simulink model "task_2"  (R2021b)
settings: Solver=VariableStepAuto  StartTime=0.0  StopTime=t  MaxStep=1e-2  RelTol=1e-3
values from neighbouring files (symbols this model uses):
  a1 = -4    [env_practice_2.m]
  a2 = -1.6    [env_practice_2.m]
  adapt_control = 1    [env_practice_2.m]
  am1 = -100/9    (= -11.1111111111)    [env_practice_2.m]
  am2 = -50/9    (= -5.55555555556)    [env_practice_2.m]
  b = 8    [env_practice_2.m]
  bm = 300/9    (= 33.3333333333)    [env_practice_2.m]
  ga = ga.*100    [env_practice_2.m]
  gb = gb*100    (= 100)    [env_practice_2.m]
  P = [1.34 0.045; 0.045 0.0981]    [env_practice_2.m]
  pulse = 1    [env_practice_2.m]
undefined symbols (not defined in the file or in its folder): au, bu, ga1, ga2
settings Model: Creator=79159  LastModifiedBy=79159

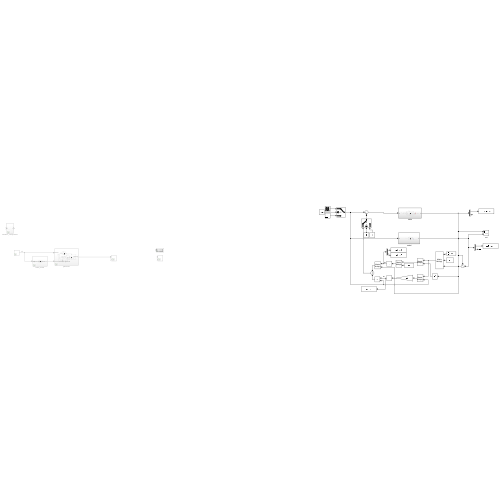
[thumbnail: Simulink's stored preview of the top-level diagram]
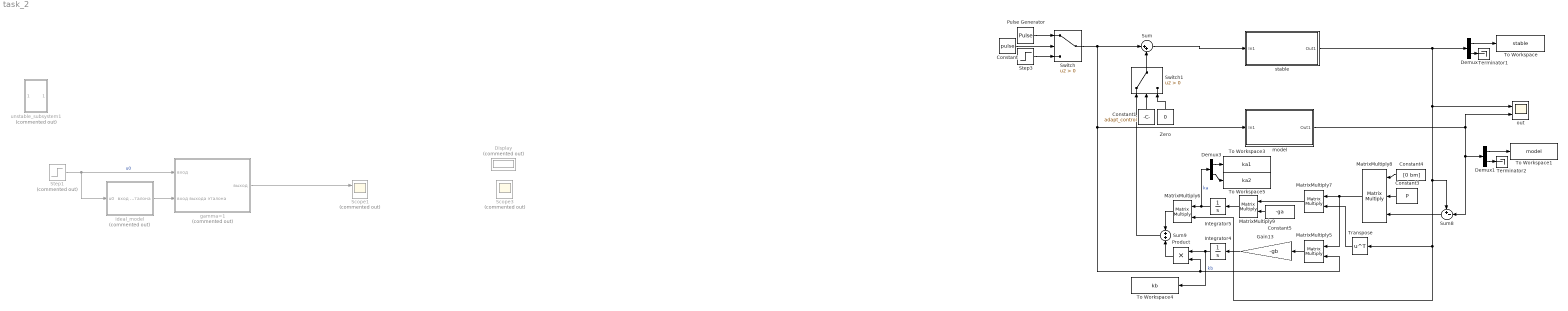
== system task_2 ==
  Constant : Constant  Value=pulse
  Constant1 : Constant  Value=adapt_control
  Constant3 : Constant  Value=P  VectorParams1D=off
  Constant4 : Constant  Value=[0 bm]  VectorParams1D=off
  Constant5 : Constant  Value=-ga  VectorParams1D=off
  Demux : Demux  Outputs=2
  Demux1 : Demux  Outputs=2
  Demux3 : Demux  Outputs=2
  Display : Display  Commented=on
      settings: Decimation=2
  Gain13 : Gain  Gain=-gb
  Integrator4 : Integrator
  Integrator5 : Integrator
  MatrixMultiply{5..7,9} (4 alike) : Product  Multiplication=Matrix(*)
  MatrixMultiply8 : Product  Inputs=3  Multiplication=Matrix(*)
  Product : Product
  Pulse Generator : DiscretePulseGenerator  PulseType=Time based  Period=20  PulseWidth=50
  Scope1 : Scope  Commented=on  NumInputPorts=2
  Scope3 : Scope  Commented=on  NumInputPorts=2
  Step1 : Step  Commented=on  Time=0  SampleTime=0
  Step3 : Step  Time=0  SampleTime=0
  Sum : Sum  Inputs=|++
  Sum8 : Sum  Inputs=+-|
  Sum9 : Sum  Inputs=+|+
  Switch : Switch  Criteria=u2 > Threshold
  Switch1 : Switch  Criteria=u2 > Threshold
  Terminator1 : Terminator
  Terminator2 : Terminator
  To Workspace : ToWorkspace  VariableName=stable  SaveFormat=Timeseries  SampleTime=-1
  To Workspace1 : ToWorkspace  VariableName=model  SaveFormat=Timeseries  SampleTime=-1
  To Workspace3 : ToWorkspace  VariableName=ka1  SaveFormat=Timeseries  SampleTime=-1
  To Workspace4 : ToWorkspace  VariableName=kb  SaveFormat=Timeseries  SampleTime=-1
  To Workspace5 : ToWorkspace  VariableName=ka2  SaveFormat=Timeseries  SampleTime=-1
  Transpose : Math  Operator=transpose  SaturateOnIntegerOverflow=on
  Zero : Constant  Value=0  OutDataTypeStr=Inherit: Inherit via back propagation
  gamma=1 : Subsystem  Commented=on
  ideal_model : Subsystem  Commented=on
  model : Subsystem
  out : Scope  NumInputPorts=2
  stable : Subsystem
  unstable_subsystem1 : Subsystem  Commented=on
  wires:
  Step1/1 -> ideal_model/1(u0), gamma=1/1(вход)  "u0"
  ideal_model/1(вход выхода эталона) -> gamma=1/2(вход выхода эталона)
  gamma=1/1(выход) -> Scope1/1
  Switch/1 -> model/1(In1), Product/2, MatrixMultiply5/2, Sum/1
  Product/1 -> Sum9/2
  stable/1(Out1) -> Demux/1, out/1, Sum8/1, Transpose/1, MatrixMultiply6/2
  MatrixMultiply7/1 -> MatrixMultiply9/1
  Sum8/1 -> MatrixMultiply8/3
  MatrixMultiply8/1 -> MatrixMultiply5/1, MatrixMultiply7/1
  Constant5/1 -> MatrixMultiply9/2
  Constant4/1 -> MatrixMultiply8/1
  Constant3/1 -> MatrixMultiply8/2
  Integrator5/1 -> Demux3/1, MatrixMultiply6/1  "ka"
  MatrixMultiply6/1 -> Sum9/1
  Gain13/1 -> Integrator4/1
  Transpose/1 -> MatrixMultiply7/2
  MatrixMultiply9/1 -> Integrator5/1
  MatrixMultiply5/1 -> Gain13/1
  Integrator4/1 -> To Workspace4/1, Product/1  "kb"
  Sum/1 -> stable/1(In1)
  model/1(Out1) -> Demux1/1, Sum8/2, out/2
  Demux/1 -> To Workspace/1
  Demux1/1 -> To Workspace1/1
  Demux3/1 -> To Workspace3/1
  Demux3/2 -> To Workspace5/1
  Demux/2 -> Terminator1/1
  Demux1/2 -> Terminator2/1
  Pulse Generator/1 -> Switch/1
  Step3/1 -> Switch/3
  Constant/1 -> Switch/2
  Sum9/1 -> Switch1/1
  Constant1/1 -> Switch1/2
  Switch1/1 -> Sum/2
  Zero/1 -> Switch1/3

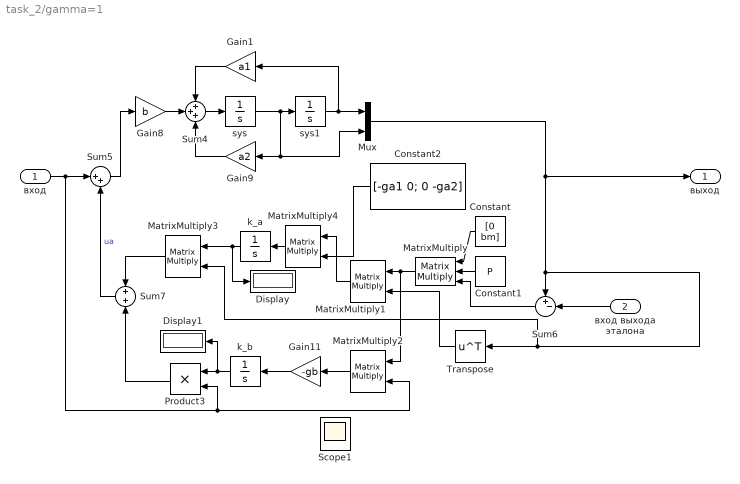
== system task_2/gamma=1 ==
  вход : Inport
  вход выхода эталона : Inport  Port=2
  Constant : Constant  Value=[0 bm]
  Constant1 : Constant  Value=P
  Constant2 : Constant  Value=[-ga1 0; 0 -ga2]
  Display : Display
      settings: Decimation=2
  Display1 : Display
      settings: Decimation=2
  Gain1 : Gain  Gain=a1
  Gain11 : Gain  Gain=-gb
  Gain8 : Gain  Gain=b
  Gain9 : Gain  Gain=a2
  MatrixMultiply : Product  Inputs=3  Multiplication=Matrix(*)
  MatrixMultiply{1..4} (4 alike) : Product  Multiplication=Matrix(*)
  Mux : Mux  Inputs=2
  Product3 : Product
  Scope1 : Scope  NumInputPorts=2
  Sum4 : Sum  Inputs=+++
  Sum5 : Sum  Inputs=|++
  Sum6 : Sum  Inputs=+-|
  Sum7 : Sum
  Transpose : Math  Operator=transpose  SaturateOnIntegerOverflow=on
  k_a : Integrator
  k_b : Integrator
  sys : Integrator
  sys1 : Integrator
  выход : Outport
  wires:
  Product3/1 -> Sum7/2
  k_b/1 -> Display1/1, Product3/1
  Sum7/1 -> Sum5/2  "ua"
  вход/1 -> MatrixMultiply2/2, Product3/2, Sum5/1
  Mux/1 -> MatrixMultiply3/2, Transpose/1, Sum6/1, выход/1
  Constant/1 -> MatrixMultiply/1
  MatrixMultiply2/1 -> Gain11/1
  MatrixMultiply3/1 -> Sum7/1
  Gain11/1 -> k_b/1
  MatrixMultiply/1 -> MatrixMultiply2/1, MatrixMultiply1/1
  вход выхода эталона/1 -> Sum6/2
  Constant1/1 -> MatrixMultiply/2
  Sum6/1 -> MatrixMultiply/3
  Transpose/1 -> MatrixMultiply1/2
  k_a/1 -> MatrixMultiply3/1, Display/1
  MatrixMultiply4/1 -> k_a/1
  MatrixMultiply1/1 -> MatrixMultiply4/1
  Constant2/1 -> MatrixMultiply4/2
  sys1/1 -> Mux/1, Gain1/1
  Sum4/1 -> sys/1
  Gain8/1 -> Sum4/2
  Gain9/1 -> Sum4/3
  sys/1 -> Mux/2, Gain9/1, sys1/1
  Sum5/1 -> Gain8/1
  Gain1/1 -> Sum4/1

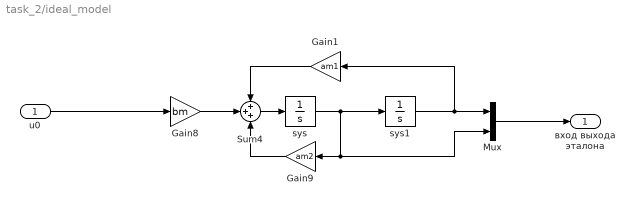
== system task_2/ideal_model ==
  u0 : Inport
  Gain1 : Gain  Gain=am1
  Gain8 : Gain  Gain=bm
  Gain9 : Gain  Gain=am2
  Mux : Mux  Inputs=2
  Sum4 : Sum  Inputs=+++
  sys : Integrator
  sys1 : Integrator
  вход выхода эталона : Outport
  wires:
  Mux/1 -> вход выхода эталона/1
  Gain9/1 -> Sum4/3
  Gain8/1 -> Sum4/2
  Sum4/1 -> sys/1
  sys/1 -> sys1/1, Gain9/1, Mux/2
  u0/1 -> Gain8/1
  sys1/1 -> Gain1/1, Mux/1
  Gain1/1 -> Sum4/1

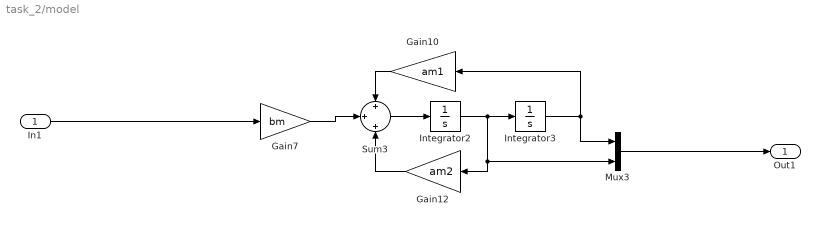
== system task_2/model ==
  In1 : Inport
  Gain10 : Gain  Gain=am1
  Gain12 : Gain  Gain=am2
  Gain7 : Gain  Gain=bm
  Integrator2 : Integrator
  Integrator3 : Integrator
  Mux3 : Mux  Inputs=2
  Sum3 : Sum  Inputs=+|+|+
  Out1 : Outport
  wires:
  In1/1 -> Gain7/1
  Sum3/1 -> Integrator2/1
  Integrator3/1 -> Mux3/1, Gain10/1
  Gain12/1 -> Sum3/3
  Gain7/1 -> Sum3/2
  Mux3/1 -> Out1/1
  Gain10/1 -> Sum3/1
  Integrator2/1 -> Integrator3/1, Gain12/1, Mux3/2

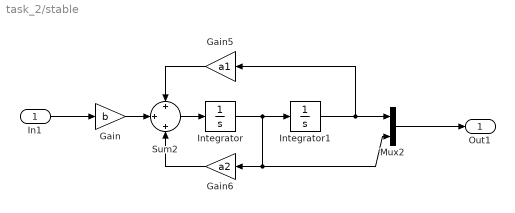
== system task_2/stable ==
  In1 : Inport
  Gain : Gain  Gain=b
  Gain5 : Gain  Gain=a1
  Gain6 : Gain  Gain=a2
  Integrator : Integrator
  Integrator1 : Integrator
  Mux2 : Mux  Inputs=2
  Sum2 : Sum  Inputs=+|+|+
  Out1 : Outport
  wires:
  Integrator/1 -> Gain6/1, Mux2/2, Integrator1/1
  Sum2/1 -> Integrator/1
  Integrator1/1 -> Mux2/1, Gain5/1
  Gain/1 -> Sum2/2
  Gain6/1 -> Sum2/3
  In1/1 -> Gain/1
  Gain5/1 -> Sum2/1
  Mux2/1 -> Out1/1

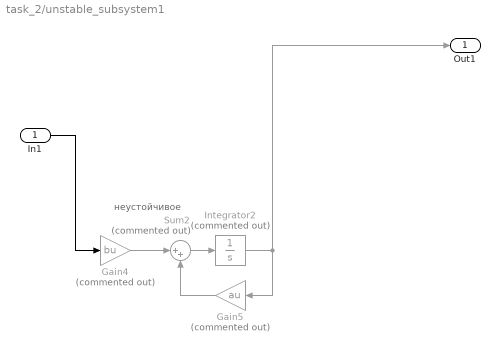
== system task_2/unstable_subsystem1 ==
  note: неустойчивое
  In1 : Inport
  Gain4 : Gain  Commented=on  Gain=bu
  Gain5 : Gain  Commented=on  Gain=au
  Integrator2 : Integrator  Commented=on
  Sum2 : Sum  Commented=on  Inputs=|++
  Out1 : Outport
  wires:
  Gain4/1 -> Sum2/1
  Sum2/1 -> Integrator2/1
  In1/1 -> Gain4/1
  Gain5/1 -> Sum2/2
  Integrator2/1 -> Gain5/1, Out1/1
